simulink model "aavs1_8ap"  (R2013a)
settings: Solver=ode45  StartTime=0.0  StopTime=10.0  RelTol=1e-3
undefined symbols (not defined in the file or in its folder): sfp
libraries: xbsIndex_r4 x1437, casper_library_misc x32, xps_library x17
(part 3 of 11)

== system aavs1_8ap/eq/quant13 ==
  cin : Inport
  din : Inport  Port=2
  Delay{,1..3} (4 alike) : xbsIndex_r4/Delay  rst=off  infoeditControl=Selection of Reset will increase slice count due to use of real FFs and instead of SRLs  en=off  latency=1  dbl_ovrd=off  reg_retiming=off  block_type=delay
  Mult : xbsIndex_r4/Mult  precision=Full  arith_type="Signed  (2's comp)"  n_bits=16  bin_pt=14  quantization=Truncate  overflow=Wrap  en=off  latency=3  dbl_ovrd=off  use_behavioral_HDL=off  opt=Speed  use_embedded=on  optimum_pipeline=off  pipeline=on  use_rpm=on  placement_style=Triangular  block_type=mult
  Mult1 : xbsIndex_r4/Mult  precision=Full  arith_type="Signed  (2's comp)"  n_bits=16  bin_pt=14  quantization=Truncate  overflow=Wrap  en=off  latency=3  dbl_ovrd=off  use_behavioral_HDL=off  opt=Speed  use_embedded=on  optimum_pipeline=off  pipeline=on  use_rpm=on  placement_style=Triangular  block_type=mult
  and : xbsIndex_r4/Logical  logical_function=OR  inputs=2  en=off  latency=1  precision=Full  arith_type=Unsigned  n_bits=16  bin_pt=0  align_bp=on  dbl_ovrd=off  block_type=logical
  c_to_ri : casper_library_misc/c_to_ri  n_bits=18  bin_pt=17
  convert_of : Subsystem  AncestorBlock=casper_library_misc/convert_of  mask(convert_of){bit_width_i=16+18, binary_point_i=17+8, bit_width_o=8, binary_point_o=7, latency=3, adder_imp=DSP48, overflow=Saturate, quantization=Round  (unbiased: even values)}
      mask prompts: bit_width_i "Bit Width In"; binary_point_i "Binary Point In"; bit_width_o "Bit Width Out"; binary_point_o "Binary Point Out"; adder_imp "Adder Implementation"; overflow "Overflow Behaviour"; quantization "Quantization Behaviour"
      mask help:
      | Converts from one 2's complement bit-width
      | and/or binary point position to another.
      | Includes underflow/overflow indicator.
      mask init: same as aavs1_8ap/eq/quant/convert_of
      settings: AttributesFormatString=[34,25]->[8,7]
      mask TypeOptions adder_imp: Fabric | DSP48
      mask TypeOptions overflow: Wrap | Saturate | Error
      mask TypeOptions quantization: Truncate | Round  (unbiased: +/- Inf) | Round  (unbiased: even values)
  convert_of1 : Subsystem  AncestorBlock=casper_library_misc/convert_of  mask(convert_of){bit_width_i=16+18, binary_point_i=17+8, bit_width_o=8, binary_point_o=7, latency=3, adder_imp=DSP48, overflow=Saturate, quantization=Round  (unbiased: even values)}
      mask prompts: bit_width_i "Bit Width In"; binary_point_i "Binary Point In"; bit_width_o "Bit Width Out"; binary_point_o "Binary Point Out"; adder_imp "Adder Implementation"; overflow "Overflow Behaviour"; quantization "Quantization Behaviour"
      mask help:
      | Converts from one 2's complement bit-width
      | and/or binary point position to another.
      | Includes underflow/overflow indicator.
      mask init: same as aavs1_8ap/eq/quant/convert_of
      settings: AttributesFormatString=[34,25]->[8,7]
      mask TypeOptions adder_imp: Fabric | DSP48
      mask TypeOptions overflow: Wrap | Saturate | Error
      mask TypeOptions quantization: Truncate | Round  (unbiased: +/- Inf) | Round  (unbiased: even values)
  ri_to_c : casper_library_misc/ri_to_c
  symmetrize : Subsystem
  symmetrize1 : Subsystem
  dout : Outport
  of : Outport  Port=2
  wires:
  c_to_ri/2 -> Mult1/2
  c_to_ri/1 -> Mult/2
  symmetrize1/1(dout) -> ri_to_c/2
  symmetrize/1(dout) -> ri_to_c/1
  convert_of/1(dout) -> Delay2/1
  convert_of1/1(dout) -> Delay3/1
  Mult1/1 -> Delay/1
  convert_of1/2(of) -> and/2
  Mult/1 -> Delay1/1
  din/1 -> c_to_ri/1
  convert_of/2(of) -> and/1
  cin/1 -> Mult1/1, Mult/1
  and/1 -> of/1
  ri_to_c/1 -> dout/1
  Delay/1 -> convert_of1/1(din)
  Delay1/1 -> convert_of/1(din)
  Delay2/1 -> symmetrize/1(din)
  Delay3/1 -> symmetrize1/1(din)

== system aavs1_8ap/eq/quant14 ==
  cin : Inport
  din : Inport  Port=2
  Delay{,1..3} (4 alike) : xbsIndex_r4/Delay  rst=off  infoeditControl=Selection of Reset will increase slice count due to use of real FFs and instead of SRLs  en=off  latency=1  dbl_ovrd=off  reg_retiming=off  block_type=delay
  Mult : xbsIndex_r4/Mult  precision=Full  arith_type="Signed  (2's comp)"  n_bits=16  bin_pt=14  quantization=Truncate  overflow=Wrap  en=off  latency=3  dbl_ovrd=off  use_behavioral_HDL=off  opt=Speed  use_embedded=on  optimum_pipeline=off  pipeline=on  use_rpm=on  placement_style=Triangular  block_type=mult
  Mult1 : xbsIndex_r4/Mult  precision=Full  arith_type="Signed  (2's comp)"  n_bits=16  bin_pt=14  quantization=Truncate  overflow=Wrap  en=off  latency=3  dbl_ovrd=off  use_behavioral_HDL=off  opt=Speed  use_embedded=on  optimum_pipeline=off  pipeline=on  use_rpm=on  placement_style=Triangular  block_type=mult
  and : xbsIndex_r4/Logical  logical_function=OR  inputs=2  en=off  latency=1  precision=Full  arith_type=Unsigned  n_bits=16  bin_pt=0  align_bp=on  dbl_ovrd=off  block_type=logical
  c_to_ri : casper_library_misc/c_to_ri  n_bits=18  bin_pt=17
  convert_of : Subsystem  AncestorBlock=casper_library_misc/convert_of  mask(convert_of){bit_width_i=16+18, binary_point_i=17+8, bit_width_o=8, binary_point_o=7, latency=3, adder_imp=DSP48, overflow=Saturate, quantization=Round  (unbiased: even values)}
      mask prompts: bit_width_i "Bit Width In"; binary_point_i "Binary Point In"; bit_width_o "Bit Width Out"; binary_point_o "Binary Point Out"; adder_imp "Adder Implementation"; overflow "Overflow Behaviour"; quantization "Quantization Behaviour"
      mask help:
      | Converts from one 2's complement bit-width
      | and/or binary point position to another.
      | Includes underflow/overflow indicator.
      mask init: same as aavs1_8ap/eq/quant/convert_of
      settings: AttributesFormatString=[34,25]->[8,7]
      mask TypeOptions adder_imp: Fabric | DSP48
      mask TypeOptions overflow: Wrap | Saturate | Error
      mask TypeOptions quantization: Truncate | Round  (unbiased: +/- Inf) | Round  (unbiased: even values)
  convert_of1 : Subsystem  AncestorBlock=casper_library_misc/convert_of  mask(convert_of){bit_width_i=16+18, binary_point_i=17+8, bit_width_o=8, binary_point_o=7, latency=3, adder_imp=DSP48, overflow=Saturate, quantization=Round  (unbiased: even values)}
      mask prompts: bit_width_i "Bit Width In"; binary_point_i "Binary Point In"; bit_width_o "Bit Width Out"; binary_point_o "Binary Point Out"; adder_imp "Adder Implementation"; overflow "Overflow Behaviour"; quantization "Quantization Behaviour"
      mask help:
      | Converts from one 2's complement bit-width
      | and/or binary point position to another.
      | Includes underflow/overflow indicator.
      mask init: same as aavs1_8ap/eq/quant/convert_of
      settings: AttributesFormatString=[34,25]->[8,7]
      mask TypeOptions adder_imp: Fabric | DSP48
      mask TypeOptions overflow: Wrap | Saturate | Error
      mask TypeOptions quantization: Truncate | Round  (unbiased: +/- Inf) | Round  (unbiased: even values)
  ri_to_c : casper_library_misc/ri_to_c
  symmetrize : Subsystem
  symmetrize1 : Subsystem
  dout : Outport
  of : Outport  Port=2
  wires:
  Delay3/1 -> symmetrize1/1(din)
  Delay2/1 -> symmetrize/1(din)
  Delay1/1 -> convert_of/1(din)
  Delay/1 -> convert_of1/1(din)
  ri_to_c/1 -> dout/1
  and/1 -> of/1
  cin/1 -> Mult/1, Mult1/1
  convert_of/2(of) -> and/1
  din/1 -> c_to_ri/1
  Mult/1 -> Delay1/1
  convert_of1/2(of) -> and/2
  Mult1/1 -> Delay/1
  convert_of1/1(dout) -> Delay3/1
  convert_of/1(dout) -> Delay2/1
  symmetrize/1(dout) -> ri_to_c/1
  symmetrize1/1(dout) -> ri_to_c/2
  c_to_ri/1 -> Mult/2
  c_to_ri/2 -> Mult1/2

== system aavs1_8ap/eq/quant15 ==
  cin : Inport
  din : Inport  Port=2
  Delay{,1..3} (4 alike) : xbsIndex_r4/Delay  rst=off  infoeditControl=Selection of Reset will increase slice count due to use of real FFs and instead of SRLs  en=off  latency=1  dbl_ovrd=off  reg_retiming=off  block_type=delay
  Mult : xbsIndex_r4/Mult  precision=Full  arith_type="Signed  (2's comp)"  n_bits=16  bin_pt=14  quantization=Truncate  overflow=Wrap  en=off  latency=3  dbl_ovrd=off  use_behavioral_HDL=off  opt=Speed  use_embedded=on  optimum_pipeline=off  pipeline=on  use_rpm=on  placement_style=Triangular  block_type=mult
  Mult1 : xbsIndex_r4/Mult  precision=Full  arith_type="Signed  (2's comp)"  n_bits=16  bin_pt=14  quantization=Truncate  overflow=Wrap  en=off  latency=3  dbl_ovrd=off  use_behavioral_HDL=off  opt=Speed  use_embedded=on  optimum_pipeline=off  pipeline=on  use_rpm=on  placement_style=Triangular  block_type=mult
  and : xbsIndex_r4/Logical  logical_function=OR  inputs=2  en=off  latency=1  precision=Full  arith_type=Unsigned  n_bits=16  bin_pt=0  align_bp=on  dbl_ovrd=off  block_type=logical
  c_to_ri : casper_library_misc/c_to_ri  n_bits=18  bin_pt=17
  convert_of : Subsystem  AncestorBlock=casper_library_misc/convert_of  mask(convert_of){bit_width_i=16+18, binary_point_i=17+8, bit_width_o=8, binary_point_o=7, latency=3, adder_imp=DSP48, overflow=Saturate, quantization=Round  (unbiased: even values)}
      mask prompts: bit_width_i "Bit Width In"; binary_point_i "Binary Point In"; bit_width_o "Bit Width Out"; binary_point_o "Binary Point Out"; adder_imp "Adder Implementation"; overflow "Overflow Behaviour"; quantization "Quantization Behaviour"
      mask help:
      | Converts from one 2's complement bit-width
      | and/or binary point position to another.
      | Includes underflow/overflow indicator.
      mask init: same as aavs1_8ap/eq/quant/convert_of
      settings: AttributesFormatString=[34,25]->[8,7]
      mask TypeOptions adder_imp: Fabric | DSP48
      mask TypeOptions overflow: Wrap | Saturate | Error
      mask TypeOptions quantization: Truncate | Round  (unbiased: +/- Inf) | Round  (unbiased: even values)
  convert_of1 : Subsystem  AncestorBlock=casper_library_misc/convert_of  mask(convert_of){bit_width_i=16+18, binary_point_i=17+8, bit_width_o=8, binary_point_o=7, latency=3, adder_imp=DSP48, overflow=Saturate, quantization=Round  (unbiased: even values)}
      mask prompts: bit_width_i "Bit Width In"; binary_point_i "Binary Point In"; bit_width_o "Bit Width Out"; binary_point_o "Binary Point Out"; adder_imp "Adder Implementation"; overflow "Overflow Behaviour"; quantization "Quantization Behaviour"
      mask help:
      | Converts from one 2's complement bit-width
      | and/or binary point position to another.
      | Includes underflow/overflow indicator.
      mask init: same as aavs1_8ap/eq/quant/convert_of
      settings: AttributesFormatString=[34,25]->[8,7]
      mask TypeOptions adder_imp: Fabric | DSP48
      mask TypeOptions overflow: Wrap | Saturate | Error
      mask TypeOptions quantization: Truncate | Round  (unbiased: +/- Inf) | Round  (unbiased: even values)
  ri_to_c : casper_library_misc/ri_to_c
  symmetrize : Subsystem
  symmetrize1 : Subsystem
  dout : Outport
  of : Outport  Port=2
  wires:
  c_to_ri/2 -> Mult1/2
  c_to_ri/1 -> Mult/2
  symmetrize1/1(dout) -> ri_to_c/2
  symmetrize/1(dout) -> ri_to_c/1
  convert_of/1(dout) -> Delay2/1
  convert_of1/1(dout) -> Delay3/1
  Mult1/1 -> Delay/1
  convert_of1/2(of) -> and/2
  Mult/1 -> Delay1/1
  din/1 -> c_to_ri/1
  convert_of/2(of) -> and/1
  cin/1 -> Mult1/1, Mult/1
  and/1 -> of/1
  ri_to_c/1 -> dout/1
  Delay/1 -> convert_of1/1(din)
  Delay1/1 -> convert_of/1(din)
  Delay2/1 -> symmetrize/1(din)
  Delay3/1 -> symmetrize1/1(din)

== system aavs1_8ap/eq/quant2 ==
  cin : Inport
  din : Inport  Port=2
  Delay{,1..3} (4 alike) : xbsIndex_r4/Delay  rst=off  infoeditControl=Selection of Reset will increase slice count due to use of real FFs and instead of SRLs  en=off  latency=1  dbl_ovrd=off  reg_retiming=off  block_type=delay
  Mult : xbsIndex_r4/Mult  precision=Full  arith_type="Signed  (2's comp)"  n_bits=16  bin_pt=14  quantization=Truncate  overflow=Wrap  en=off  latency=3  dbl_ovrd=off  use_behavioral_HDL=off  opt=Speed  use_embedded=on  optimum_pipeline=off  pipeline=on  use_rpm=on  placement_style=Triangular  block_type=mult
  Mult1 : xbsIndex_r4/Mult  precision=Full  arith_type="Signed  (2's comp)"  n_bits=16  bin_pt=14  quantization=Truncate  overflow=Wrap  en=off  latency=3  dbl_ovrd=off  use_behavioral_HDL=off  opt=Speed  use_embedded=on  optimum_pipeline=off  pipeline=on  use_rpm=on  placement_style=Triangular  block_type=mult
  and : xbsIndex_r4/Logical  logical_function=OR  inputs=2  en=off  latency=1  precision=Full  arith_type=Unsigned  n_bits=16  bin_pt=0  align_bp=on  dbl_ovrd=off  block_type=logical
  c_to_ri : casper_library_misc/c_to_ri  n_bits=18  bin_pt=17
  convert_of : Subsystem  AncestorBlock=casper_library_misc/convert_of  mask(convert_of){bit_width_i=16+18, binary_point_i=17+8, bit_width_o=8, binary_point_o=7, latency=3, adder_imp=DSP48, overflow=Saturate, quantization=Round  (unbiased: even values)}
      mask prompts: bit_width_i "Bit Width In"; binary_point_i "Binary Point In"; bit_width_o "Bit Width Out"; binary_point_o "Binary Point Out"; adder_imp "Adder Implementation"; overflow "Overflow Behaviour"; quantization "Quantization Behaviour"
      mask help:
      | Converts from one 2's complement bit-width
      | and/or binary point position to another.
      | Includes underflow/overflow indicator.
      mask init: same as aavs1_8ap/eq/quant/convert_of
      settings: AttributesFormatString=[34,25]->[8,7]
      mask TypeOptions adder_imp: Fabric | DSP48
      mask TypeOptions overflow: Wrap | Saturate | Error
      mask TypeOptions quantization: Truncate | Round  (unbiased: +/- Inf) | Round  (unbiased: even values)
  convert_of1 : Subsystem  AncestorBlock=casper_library_misc/convert_of  mask(convert_of){bit_width_i=16+18, binary_point_i=17+8, bit_width_o=8, binary_point_o=7, latency=3, adder_imp=DSP48, overflow=Saturate, quantization=Round  (unbiased: even values)}
      mask prompts: bit_width_i "Bit Width In"; binary_point_i "Binary Point In"; bit_width_o "Bit Width Out"; binary_point_o "Binary Point Out"; adder_imp "Adder Implementation"; overflow "Overflow Behaviour"; quantization "Quantization Behaviour"
      mask help:
      | Converts from one 2's complement bit-width
      | and/or binary point position to another.
      | Includes underflow/overflow indicator.
      mask init: same as aavs1_8ap/eq/quant/convert_of
      settings: AttributesFormatString=[34,25]->[8,7]
      mask TypeOptions adder_imp: Fabric | DSP48
      mask TypeOptions overflow: Wrap | Saturate | Error
      mask TypeOptions quantization: Truncate | Round  (unbiased: +/- Inf) | Round  (unbiased: even values)
  ri_to_c : casper_library_misc/ri_to_c
  symmetrize : Subsystem
  symmetrize1 : Subsystem
  dout : Outport
  of : Outport  Port=2
  wires:
  c_to_ri/2 -> Mult1/2
  c_to_ri/1 -> Mult/2
  symmetrize1/1(dout) -> ri_to_c/2
  symmetrize/1(dout) -> ri_to_c/1
  convert_of/1(dout) -> Delay2/1
  convert_of1/1(dout) -> Delay3/1
  Mult1/1 -> Delay/1
  convert_of1/2(of) -> and/2
  Mult/1 -> Delay1/1
  din/1 -> c_to_ri/1
  convert_of/2(of) -> and/1
  cin/1 -> Mult1/1, Mult/1
  and/1 -> of/1
  ri_to_c/1 -> dout/1
  Delay/1 -> convert_of1/1(din)
  Delay1/1 -> convert_of/1(din)
  Delay2/1 -> symmetrize/1(din)
  Delay3/1 -> symmetrize1/1(din)

== system aavs1_8ap/eq/quant3 ==
  cin : Inport
  din : Inport  Port=2
  Delay{,1..3} (4 alike) : xbsIndex_r4/Delay  rst=off  infoeditControl=Selection of Reset will increase slice count due to use of real FFs and instead of SRLs  en=off  latency=1  dbl_ovrd=off  reg_retiming=off  block_type=delay
  Mult : xbsIndex_r4/Mult  precision=Full  arith_type="Signed  (2's comp)"  n_bits=16  bin_pt=14  quantization=Truncate  overflow=Wrap  en=off  latency=3  dbl_ovrd=off  use_behavioral_HDL=off  opt=Speed  use_embedded=on  optimum_pipeline=off  pipeline=on  use_rpm=on  placement_style=Triangular  block_type=mult
  Mult1 : xbsIndex_r4/Mult  precision=Full  arith_type="Signed  (2's comp)"  n_bits=16  bin_pt=14  quantization=Truncate  overflow=Wrap  en=off  latency=3  dbl_ovrd=off  use_behavioral_HDL=off  opt=Speed  use_embedded=on  optimum_pipeline=off  pipeline=on  use_rpm=on  placement_style=Triangular  block_type=mult
  and : xbsIndex_r4/Logical  logical_function=OR  inputs=2  en=off  latency=1  precision=Full  arith_type=Unsigned  n_bits=16  bin_pt=0  align_bp=on  dbl_ovrd=off  block_type=logical
  c_to_ri : casper_library_misc/c_to_ri  n_bits=18  bin_pt=17
  convert_of : Subsystem  AncestorBlock=casper_library_misc/convert_of  mask(convert_of){bit_width_i=16+18, binary_point_i=17+8, bit_width_o=8, binary_point_o=7, latency=3, adder_imp=DSP48, overflow=Saturate, quantization=Round  (unbiased: even values)}
      mask prompts: bit_width_i "Bit Width In"; binary_point_i "Binary Point In"; bit_width_o "Bit Width Out"; binary_point_o "Binary Point Out"; adder_imp "Adder Implementation"; overflow "Overflow Behaviour"; quantization "Quantization Behaviour"
      mask help:
      | Converts from one 2's complement bit-width
      | and/or binary point position to another.
      | Includes underflow/overflow indicator.
      mask init: same as aavs1_8ap/eq/quant/convert_of
      settings: AttributesFormatString=[34,25]->[8,7]
      mask TypeOptions adder_imp: Fabric | DSP48
      mask TypeOptions overflow: Wrap | Saturate | Error
      mask TypeOptions quantization: Truncate | Round  (unbiased: +/- Inf) | Round  (unbiased: even values)
  convert_of1 : Subsystem  AncestorBlock=casper_library_misc/convert_of  mask(convert_of){bit_width_i=16+18, binary_point_i=17+8, bit_width_o=8, binary_point_o=7, latency=3, adder_imp=DSP48, overflow=Saturate, quantization=Round  (unbiased: even values)}
      mask prompts: bit_width_i "Bit Width In"; binary_point_i "Binary Point In"; bit_width_o "Bit Width Out"; binary_point_o "Binary Point Out"; adder_imp "Adder Implementation"; overflow "Overflow Behaviour"; quantization "Quantization Behaviour"
      mask help:
      | Converts from one 2's complement bit-width
      | and/or binary point position to another.
      | Includes underflow/overflow indicator.
      mask init: same as aavs1_8ap/eq/quant/convert_of
      settings: AttributesFormatString=[34,25]->[8,7]
      mask TypeOptions adder_imp: Fabric | DSP48
      mask TypeOptions overflow: Wrap | Saturate | Error
      mask TypeOptions quantization: Truncate | Round  (unbiased: +/- Inf) | Round  (unbiased: even values)
  ri_to_c : casper_library_misc/ri_to_c
  symmetrize : Subsystem
  symmetrize1 : Subsystem
  dout : Outport
  of : Outport  Port=2
  wires:
  Delay3/1 -> symmetrize1/1(din)
  Delay2/1 -> symmetrize/1(din)
  Delay1/1 -> convert_of/1(din)
  Delay/1 -> convert_of1/1(din)
  ri_to_c/1 -> dout/1
  and/1 -> of/1
  cin/1 -> Mult/1, Mult1/1
  convert_of/2(of) -> and/1
  din/1 -> c_to_ri/1
  Mult/1 -> Delay1/1
  convert_of1/2(of) -> and/2
  Mult1/1 -> Delay/1
  convert_of1/1(dout) -> Delay3/1
  convert_of/1(dout) -> Delay2/1
  symmetrize/1(dout) -> ri_to_c/1
  symmetrize1/1(dout) -> ri_to_c/2
  c_to_ri/1 -> Mult/2
  c_to_ri/2 -> Mult1/2

== system aavs1_8ap/eq/quant4 ==
  cin : Inport
  din : Inport  Port=2
  Delay{,1..3} (4 alike) : xbsIndex_r4/Delay  rst=off  infoeditControl=Selection of Reset will increase slice count due to use of real FFs and instead of SRLs  en=off  latency=1  dbl_ovrd=off  reg_retiming=off  block_type=delay
  Mult : xbsIndex_r4/Mult  precision=Full  arith_type="Signed  (2's comp)"  n_bits=16  bin_pt=14  quantization=Truncate  overflow=Wrap  en=off  latency=3  dbl_ovrd=off  use_behavioral_HDL=off  opt=Speed  use_embedded=on  optimum_pipeline=off  pipeline=on  use_rpm=on  placement_style=Triangular  block_type=mult
  Mult1 : xbsIndex_r4/Mult  precision=Full  arith_type="Signed  (2's comp)"  n_bits=16  bin_pt=14  quantization=Truncate  overflow=Wrap  en=off  latency=3  dbl_ovrd=off  use_behavioral_HDL=off  opt=Speed  use_embedded=on  optimum_pipeline=off  pipeline=on  use_rpm=on  placement_style=Triangular  block_type=mult
  and : xbsIndex_r4/Logical  logical_function=OR  inputs=2  en=off  latency=1  precision=Full  arith_type=Unsigned  n_bits=16  bin_pt=0  align_bp=on  dbl_ovrd=off  block_type=logical
  c_to_ri : casper_library_misc/c_to_ri  n_bits=18  bin_pt=17
  convert_of : Subsystem  AncestorBlock=casper_library_misc/convert_of  mask(convert_of){bit_width_i=16+18, binary_point_i=17+8, bit_width_o=8, binary_point_o=7, latency=3, adder_imp=DSP48, overflow=Saturate, quantization=Round  (unbiased: even values)}
      mask prompts: bit_width_i "Bit Width In"; binary_point_i "Binary Point In"; bit_width_o "Bit Width Out"; binary_point_o "Binary Point Out"; adder_imp "Adder Implementation"; overflow "Overflow Behaviour"; quantization "Quantization Behaviour"
      mask help:
      | Converts from one 2's complement bit-width
      | and/or binary point position to another.
      | Includes underflow/overflow indicator.
      mask init: same as aavs1_8ap/eq/quant/convert_of
      settings: AttributesFormatString=[34,25]->[8,7]
      mask TypeOptions adder_imp: Fabric | DSP48
      mask TypeOptions overflow: Wrap | Saturate | Error
      mask TypeOptions quantization: Truncate | Round  (unbiased: +/- Inf) | Round  (unbiased: even values)
  convert_of1 : Subsystem  AncestorBlock=casper_library_misc/convert_of  mask(convert_of){bit_width_i=16+18, binary_point_i=17+8, bit_width_o=8, binary_point_o=7, latency=3, adder_imp=DSP48, overflow=Saturate, quantization=Round  (unbiased: even values)}
      mask prompts: bit_width_i "Bit Width In"; binary_point_i "Binary Point In"; bit_width_o "Bit Width Out"; binary_point_o "Binary Point Out"; adder_imp "Adder Implementation"; overflow "Overflow Behaviour"; quantization "Quantization Behaviour"
      mask help:
      | Converts from one 2's complement bit-width
      | and/or binary point position to another.
      | Includes underflow/overflow indicator.
      mask init: same as aavs1_8ap/eq/quant/convert_of
      settings: AttributesFormatString=[34,25]->[8,7]
      mask TypeOptions adder_imp: Fabric | DSP48
      mask TypeOptions overflow: Wrap | Saturate | Error
      mask TypeOptions quantization: Truncate | Round  (unbiased: +/- Inf) | Round  (unbiased: even values)
  ri_to_c : casper_library_misc/ri_to_c
  symmetrize : Subsystem
  symmetrize1 : Subsystem
  dout : Outport
  of : Outport  Port=2
  wires:
  Delay3/1 -> symmetrize1/1(din)
  Delay2/1 -> symmetrize/1(din)
  Delay1/1 -> convert_of/1(din)
  Delay/1 -> convert_of1/1(din)
  ri_to_c/1 -> dout/1
  and/1 -> of/1
  cin/1 -> Mult/1, Mult1/1
  convert_of/2(of) -> and/1
  din/1 -> c_to_ri/1
  Mult/1 -> Delay1/1
  convert_of1/2(of) -> and/2
  Mult1/1 -> Delay/1
  convert_of1/1(dout) -> Delay3/1
  convert_of/1(dout) -> Delay2/1
  symmetrize/1(dout) -> ri_to_c/1
  symmetrize1/1(dout) -> ri_to_c/2
  c_to_ri/1 -> Mult/2
  c_to_ri/2 -> Mult1/2

== system aavs1_8ap/eq/quant5 ==
  cin : Inport
  din : Inport  Port=2
  Delay{,1..3} (4 alike) : xbsIndex_r4/Delay  rst=off  infoeditControl=Selection of Reset will increase slice count due to use of real FFs and instead of SRLs  en=off  latency=1  dbl_ovrd=off  reg_retiming=off  block_type=delay
  Mult : xbsIndex_r4/Mult  precision=Full  arith_type="Signed  (2's comp)"  n_bits=16  bin_pt=14  quantization=Truncate  overflow=Wrap  en=off  latency=3  dbl_ovrd=off  use_behavioral_HDL=off  opt=Speed  use_embedded=on  optimum_pipeline=off  pipeline=on  use_rpm=on  placement_style=Triangular  block_type=mult
  Mult1 : xbsIndex_r4/Mult  precision=Full  arith_type="Signed  (2's comp)"  n_bits=16  bin_pt=14  quantization=Truncate  overflow=Wrap  en=off  latency=3  dbl_ovrd=off  use_behavioral_HDL=off  opt=Speed  use_embedded=on  optimum_pipeline=off  pipeline=on  use_rpm=on  placement_style=Triangular  block_type=mult
  and : xbsIndex_r4/Logical  logical_function=OR  inputs=2  en=off  latency=1  precision=Full  arith_type=Unsigned  n_bits=16  bin_pt=0  align_bp=on  dbl_ovrd=off  block_type=logical
  c_to_ri : casper_library_misc/c_to_ri  n_bits=18  bin_pt=17
  convert_of : Subsystem  AncestorBlock=casper_library_misc/convert_of  mask(convert_of){bit_width_i=16+18, binary_point_i=17+8, bit_width_o=8, binary_point_o=7, latency=3, adder_imp=DSP48, overflow=Saturate, quantization=Round  (unbiased: even values)}
      mask prompts: bit_width_i "Bit Width In"; binary_point_i "Binary Point In"; bit_width_o "Bit Width Out"; binary_point_o "Binary Point Out"; adder_imp "Adder Implementation"; overflow "Overflow Behaviour"; quantization "Quantization Behaviour"
      mask help:
      | Converts from one 2's complement bit-width
      | and/or binary point position to another.
      | Includes underflow/overflow indicator.
      mask init: same as aavs1_8ap/eq/quant/convert_of
      settings: AttributesFormatString=[34,25]->[8,7]
      mask TypeOptions adder_imp: Fabric | DSP48
      mask TypeOptions overflow: Wrap | Saturate | Error
      mask TypeOptions quantization: Truncate | Round  (unbiased: +/- Inf) | Round  (unbiased: even values)
  convert_of1 : Subsystem  AncestorBlock=casper_library_misc/convert_of  mask(convert_of){bit_width_i=16+18, binary_point_i=17+8, bit_width_o=8, binary_point_o=7, latency=3, adder_imp=DSP48, overflow=Saturate, quantization=Round  (unbiased: even values)}
      mask prompts: bit_width_i "Bit Width In"; binary_point_i "Binary Point In"; bit_width_o "Bit Width Out"; binary_point_o "Binary Point Out"; adder_imp "Adder Implementation"; overflow "Overflow Behaviour"; quantization "Quantization Behaviour"
      mask help:
      | Converts from one 2's complement bit-width
      | and/or binary point position to another.
      | Includes underflow/overflow indicator.
      mask init: same as aavs1_8ap/eq/quant/convert_of
      settings: AttributesFormatString=[34,25]->[8,7]
      mask TypeOptions adder_imp: Fabric | DSP48
      mask TypeOptions overflow: Wrap | Saturate | Error
      mask TypeOptions quantization: Truncate | Round  (unbiased: +/- Inf) | Round  (unbiased: even values)
  ri_to_c : casper_library_misc/ri_to_c
  symmetrize : Subsystem
  symmetrize1 : Subsystem
  dout : Outport
  of : Outport  Port=2
  wires:
  c_to_ri/2 -> Mult1/2
  c_to_ri/1 -> Mult/2
  symmetrize1/1(dout) -> ri_to_c/2
  symmetrize/1(dout) -> ri_to_c/1
  convert_of/1(dout) -> Delay2/1
  convert_of1/1(dout) -> Delay3/1
  Mult1/1 -> Delay/1
  convert_of1/2(of) -> and/2
  Mult/1 -> Delay1/1
  din/1 -> c_to_ri/1
  convert_of/2(of) -> and/1
  cin/1 -> Mult1/1, Mult/1
  and/1 -> of/1
  ri_to_c/1 -> dout/1
  Delay/1 -> convert_of1/1(din)
  Delay1/1 -> convert_of/1(din)
  Delay2/1 -> symmetrize/1(din)
  Delay3/1 -> symmetrize1/1(din)

== system aavs1_8ap/eq/quant6 ==
  cin : Inport
  din : Inport  Port=2
  Delay{,1..3} (4 alike) : xbsIndex_r4/Delay  rst=off  infoeditControl=Selection of Reset will increase slice count due to use of real FFs and instead of SRLs  en=off  latency=1  dbl_ovrd=off  reg_retiming=off  block_type=delay
  Mult : xbsIndex_r4/Mult  precision=Full  arith_type="Signed  (2's comp)"  n_bits=16  bin_pt=14  quantization=Truncate  overflow=Wrap  en=off  latency=3  dbl_ovrd=off  use_behavioral_HDL=off  opt=Speed  use_embedded=on  optimum_pipeline=off  pipeline=on  use_rpm=on  placement_style=Triangular  block_type=mult
  Mult1 : xbsIndex_r4/Mult  precision=Full  arith_type="Signed  (2's comp)"  n_bits=16  bin_pt=14  quantization=Truncate  overflow=Wrap  en=off  latency=3  dbl_ovrd=off  use_behavioral_HDL=off  opt=Speed  use_embedded=on  optimum_pipeline=off  pipeline=on  use_rpm=on  placement_style=Triangular  block_type=mult
  and : xbsIndex_r4/Logical  logical_function=OR  inputs=2  en=off  latency=1  precision=Full  arith_type=Unsigned  n_bits=16  bin_pt=0  align_bp=on  dbl_ovrd=off  block_type=logical
  c_to_ri : casper_library_misc/c_to_ri  n_bits=18  bin_pt=17
  convert_of : Subsystem  AncestorBlock=casper_library_misc/convert_of  mask(convert_of){bit_width_i=16+18, binary_point_i=17+8, bit_width_o=8, binary_point_o=7, latency=3, adder_imp=DSP48, overflow=Saturate, quantization=Round  (unbiased: even values)}
      mask prompts: bit_width_i "Bit Width In"; binary_point_i "Binary Point In"; bit_width_o "Bit Width Out"; binary_point_o "Binary Point Out"; adder_imp "Adder Implementation"; overflow "Overflow Behaviour"; quantization "Quantization Behaviour"
      mask help:
      | Converts from one 2's complement bit-width
      | and/or binary point position to another.
      | Includes underflow/overflow indicator.
      mask init: same as aavs1_8ap/eq/quant/convert_of
      settings: AttributesFormatString=[34,25]->[8,7]
      mask TypeOptions adder_imp: Fabric | DSP48
      mask TypeOptions overflow: Wrap | Saturate | Error
      mask TypeOptions quantization: Truncate | Round  (unbiased: +/- Inf) | Round  (unbiased: even values)
  convert_of1 : Subsystem  AncestorBlock=casper_library_misc/convert_of  mask(convert_of){bit_width_i=16+18, binary_point_i=17+8, bit_width_o=8, binary_point_o=7, latency=3, adder_imp=DSP48, overflow=Saturate, quantization=Round  (unbiased: even values)}
      mask prompts: bit_width_i "Bit Width In"; binary_point_i "Binary Point In"; bit_width_o "Bit Width Out"; binary_point_o "Binary Point Out"; adder_imp "Adder Implementation"; overflow "Overflow Behaviour"; quantization "Quantization Behaviour"
      mask help:
      | Converts from one 2's complement bit-width
      | and/or binary point position to another.
      | Includes underflow/overflow indicator.
      mask init: same as aavs1_8ap/eq/quant/convert_of
      settings: AttributesFormatString=[34,25]->[8,7]
      mask TypeOptions adder_imp: Fabric | DSP48
      mask TypeOptions overflow: Wrap | Saturate | Error
      mask TypeOptions quantization: Truncate | Round  (unbiased: +/- Inf) | Round  (unbiased: even values)
  ri_to_c : casper_library_misc/ri_to_c
  symmetrize : Subsystem
  symmetrize1 : Subsystem
  dout : Outport
  of : Outport  Port=2
  wires:
  Delay3/1 -> symmetrize1/1(din)
  Delay2/1 -> symmetrize/1(din)
  Delay1/1 -> convert_of/1(din)
  Delay/1 -> convert_of1/1(din)
  ri_to_c/1 -> dout/1
  and/1 -> of/1
  cin/1 -> Mult/1, Mult1/1
  convert_of/2(of) -> and/1
  din/1 -> c_to_ri/1
  Mult/1 -> Delay1/1
  convert_of1/2(of) -> and/2
  Mult1/1 -> Delay/1
  convert_of1/1(dout) -> Delay3/1
  convert_of/1(dout) -> Delay2/1
  symmetrize/1(dout) -> ri_to_c/1
  symmetrize1/1(dout) -> ri_to_c/2
  c_to_ri/1 -> Mult/2
  c_to_ri/2 -> Mult1/2

== system aavs1_8ap/eq/quant7 ==
  cin : Inport
  din : Inport  Port=2
  Delay{,1..3} (4 alike) : xbsIndex_r4/Delay  rst=off  infoeditControl=Selection of Reset will increase slice count due to use of real FFs and instead of SRLs  en=off  latency=1  dbl_ovrd=off  reg_retiming=off  block_type=delay
  Mult : xbsIndex_r4/Mult  precision=Full  arith_type="Signed  (2's comp)"  n_bits=16  bin_pt=14  quantization=Truncate  overflow=Wrap  en=off  latency=3  dbl_ovrd=off  use_behavioral_HDL=off  opt=Speed  use_embedded=on  optimum_pipeline=off  pipeline=on  use_rpm=on  placement_style=Triangular  block_type=mult
  Mult1 : xbsIndex_r4/Mult  precision=Full  arith_type="Signed  (2's comp)"  n_bits=16  bin_pt=14  quantization=Truncate  overflow=Wrap  en=off  latency=3  dbl_ovrd=off  use_behavioral_HDL=off  opt=Speed  use_embedded=on  optimum_pipeline=off  pipeline=on  use_rpm=on  placement_style=Triangular  block_type=mult
  and : xbsIndex_r4/Logical  logical_function=OR  inputs=2  en=off  latency=1  precision=Full  arith_type=Unsigned  n_bits=16  bin_pt=0  align_bp=on  dbl_ovrd=off  block_type=logical
  c_to_ri : casper_library_misc/c_to_ri  n_bits=18  bin_pt=17
  convert_of : Subsystem  AncestorBlock=casper_library_misc/convert_of  mask(convert_of){bit_width_i=16+18, binary_point_i=17+8, bit_width_o=8, binary_point_o=7, latency=3, adder_imp=DSP48, overflow=Saturate, quantization=Round  (unbiased: even values)}
      mask prompts: bit_width_i "Bit Width In"; binary_point_i "Binary Point In"; bit_width_o "Bit Width Out"; binary_point_o "Binary Point Out"; adder_imp "Adder Implementation"; overflow "Overflow Behaviour"; quantization "Quantization Behaviour"
      mask help:
      | Converts from one 2's complement bit-width
      | and/or binary point position to another.
      | Includes underflow/overflow indicator.
      mask init: same as aavs1_8ap/eq/quant/convert_of
      settings: AttributesFormatString=[34,25]->[8,7]
      mask TypeOptions adder_imp: Fabric | DSP48
      mask TypeOptions overflow: Wrap | Saturate | Error
      mask TypeOptions quantization: Truncate | Round  (unbiased: +/- Inf) | Round  (unbiased: even values)
  convert_of1 : Subsystem  AncestorBlock=casper_library_misc/convert_of  mask(convert_of){bit_width_i=16+18, binary_point_i=17+8, bit_width_o=8, binary_point_o=7, latency=3, adder_imp=DSP48, overflow=Saturate, quantization=Round  (unbiased: even values)}
      mask prompts: bit_width_i "Bit Width In"; binary_point_i "Binary Point In"; bit_width_o "Bit Width Out"; binary_point_o "Binary Point Out"; adder_imp "Adder Implementation"; overflow "Overflow Behaviour"; quantization "Quantization Behaviour"
      mask help:
      | Converts from one 2's complement bit-width
      | and/or binary point position to another.
      | Includes underflow/overflow indicator.
      mask init: same as aavs1_8ap/eq/quant/convert_of
      settings: AttributesFormatString=[34,25]->[8,7]
      mask TypeOptions adder_imp: Fabric | DSP48
      mask TypeOptions overflow: Wrap | Saturate | Error
      mask TypeOptions quantization: Truncate | Round  (unbiased: +/- Inf) | Round  (unbiased: even values)
  ri_to_c : casper_library_misc/ri_to_c
  symmetrize : Subsystem
  symmetrize1 : Subsystem
  dout : Outport
  of : Outport  Port=2
  wires:
  c_to_ri/2 -> Mult1/2
  c_to_ri/1 -> Mult/2
  symmetrize1/1(dout) -> ri_to_c/2
  symmetrize/1(dout) -> ri_to_c/1
  convert_of/1(dout) -> Delay2/1
  convert_of1/1(dout) -> Delay3/1
  Mult1/1 -> Delay/1
  convert_of1/2(of) -> and/2
  Mult/1 -> Delay1/1
  din/1 -> c_to_ri/1
  convert_of/2(of) -> and/1
  cin/1 -> Mult1/1, Mult/1
  and/1 -> of/1
  ri_to_c/1 -> dout/1
  Delay/1 -> convert_of1/1(din)
  Delay1/1 -> convert_of/1(din)
  Delay2/1 -> symmetrize/1(din)
  Delay3/1 -> symmetrize1/1(din)

== system aavs1_8ap/eq/quant8 ==
  cin : Inport
  din : Inport  Port=2
  Delay{,1..3} (4 alike) : xbsIndex_r4/Delay  rst=off  infoeditControl=Selection of Reset will increase slice count due to use of real FFs and instead of SRLs  en=off  latency=1  dbl_ovrd=off  reg_retiming=off  block_type=delay
  Mult : xbsIndex_r4/Mult  precision=Full  arith_type="Signed  (2's comp)"  n_bits=16  bin_pt=14  quantization=Truncate  overflow=Wrap  en=off  latency=3  dbl_ovrd=off  use_behavioral_HDL=off  opt=Speed  use_embedded=on  optimum_pipeline=off  pipeline=on  use_rpm=on  placement_style=Triangular  block_type=mult
  Mult1 : xbsIndex_r4/Mult  precision=Full  arith_type="Signed  (2's comp)"  n_bits=16  bin_pt=14  quantization=Truncate  overflow=Wrap  en=off  latency=3  dbl_ovrd=off  use_behavioral_HDL=off  opt=Speed  use_embedded=on  optimum_pipeline=off  pipeline=on  use_rpm=on  placement_style=Triangular  block_type=mult
  and : xbsIndex_r4/Logical  logical_function=OR  inputs=2  en=off  latency=1  precision=Full  arith_type=Unsigned  n_bits=16  bin_pt=0  align_bp=on  dbl_ovrd=off  block_type=logical
  c_to_ri : casper_library_misc/c_to_ri  n_bits=18  bin_pt=17
  convert_of : Subsystem  AncestorBlock=casper_library_misc/convert_of  mask(convert_of){bit_width_i=16+18, binary_point_i=17+8, bit_width_o=8, binary_point_o=7, latency=3, adder_imp=DSP48, overflow=Saturate, quantization=Round  (unbiased: even values)}
      mask prompts: bit_width_i "Bit Width In"; binary_point_i "Binary Point In"; bit_width_o "Bit Width Out"; binary_point_o "Binary Point Out"; adder_imp "Adder Implementation"; overflow "Overflow Behaviour"; quantization "Quantization Behaviour"
      mask help:
      | Converts from one 2's complement bit-width
      | and/or binary point position to another.
      | Includes underflow/overflow indicator.
      mask init: same as aavs1_8ap/eq/quant/convert_of
      settings: AttributesFormatString=[34,25]->[8,7]
      mask TypeOptions adder_imp: Fabric | DSP48
      mask TypeOptions overflow: Wrap | Saturate | Error
      mask TypeOptions quantization: Truncate | Round  (unbiased: +/- Inf) | Round  (unbiased: even values)
  convert_of1 : Subsystem  AncestorBlock=casper_library_misc/convert_of  mask(convert_of){bit_width_i=16+18, binary_point_i=17+8, bit_width_o=8, binary_point_o=7, latency=3, adder_imp=DSP48, overflow=Saturate, quantization=Round  (unbiased: even values)}
      mask prompts: bit_width_i "Bit Width In"; binary_point_i "Binary Point In"; bit_width_o "Bit Width Out"; binary_point_o "Binary Point Out"; adder_imp "Adder Implementation"; overflow "Overflow Behaviour"; quantization "Quantization Behaviour"
      mask help:
      | Converts from one 2's complement bit-width
      | and/or binary point position to another.
      | Includes underflow/overflow indicator.
      mask init: same as aavs1_8ap/eq/quant/convert_of
      settings: AttributesFormatString=[34,25]->[8,7]
      mask TypeOptions adder_imp: Fabric | DSP48
      mask TypeOptions overflow: Wrap | Saturate | Error
      mask TypeOptions quantization: Truncate | Round  (unbiased: +/- Inf) | Round  (unbiased: even values)
  ri_to_c : casper_library_misc/ri_to_c
  symmetrize : Subsystem
  symmetrize1 : Subsystem
  dout : Outport
  of : Outport  Port=2
  wires:
  c_to_ri/2 -> Mult1/2
  c_to_ri/1 -> Mult/2
  symmetrize1/1(dout) -> ri_to_c/2
  symmetrize/1(dout) -> ri_to_c/1
  convert_of/1(dout) -> Delay2/1
  convert_of1/1(dout) -> Delay3/1
  Mult1/1 -> Delay/1
  convert_of1/2(of) -> and/2
  Mult/1 -> Delay1/1
  din/1 -> c_to_ri/1
  convert_of/2(of) -> and/1
  cin/1 -> Mult1/1, Mult/1
  and/1 -> of/1
  ri_to_c/1 -> dout/1
  Delay/1 -> convert_of1/1(din)
  Delay1/1 -> convert_of/1(din)
  Delay2/1 -> symmetrize/1(din)
  Delay3/1 -> symmetrize1/1(din)

== system aavs1_8ap/eq/quant9 ==
  cin : Inport
  din : Inport  Port=2
  Delay{,1..3} (4 alike) : xbsIndex_r4/Delay  rst=off  infoeditControl=Selection of Reset will increase slice count due to use of real FFs and instead of SRLs  en=off  latency=1  dbl_ovrd=off  reg_retiming=off  block_type=delay
  Mult : xbsIndex_r4/Mult  precision=Full  arith_type="Signed  (2's comp)"  n_bits=16  bin_pt=14  quantization=Truncate  overflow=Wrap  en=off  latency=3  dbl_ovrd=off  use_behavioral_HDL=off  opt=Speed  use_embedded=on  optimum_pipeline=off  pipeline=on  use_rpm=on  placement_style=Triangular  block_type=mult
  Mult1 : xbsIndex_r4/Mult  precision=Full  arith_type="Signed  (2's comp)"  n_bits=16  bin_pt=14  quantization=Truncate  overflow=Wrap  en=off  latency=3  dbl_ovrd=off  use_behavioral_HDL=off  opt=Speed  use_embedded=on  optimum_pipeline=off  pipeline=on  use_rpm=on  placement_style=Triangular  block_type=mult
  and : xbsIndex_r4/Logical  logical_function=OR  inputs=2  en=off  latency=1  precision=Full  arith_type=Unsigned  n_bits=16  bin_pt=0  align_bp=on  dbl_ovrd=off  block_type=logical
  c_to_ri : casper_library_misc/c_to_ri  n_bits=18  bin_pt=17
  convert_of : Subsystem  AncestorBlock=casper_library_misc/convert_of  mask(convert_of){bit_width_i=16+18, binary_point_i=17+8, bit_width_o=8, binary_point_o=7, latency=3, adder_imp=DSP48, overflow=Saturate, quantization=Round  (unbiased: even values)}
      mask prompts: bit_width_i "Bit Width In"; binary_point_i "Binary Point In"; bit_width_o "Bit Width Out"; binary_point_o "Binary Point Out"; adder_imp "Adder Implementation"; overflow "Overflow Behaviour"; quantization "Quantization Behaviour"
      mask help:
      | Converts from one 2's complement bit-width
      | and/or binary point position to another.
      | Includes underflow/overflow indicator.
      mask init: same as aavs1_8ap/eq/quant/convert_of
      settings: AttributesFormatString=[34,25]->[8,7]
      mask TypeOptions adder_imp: Fabric | DSP48
      mask TypeOptions overflow: Wrap | Saturate | Error
      mask TypeOptions quantization: Truncate | Round  (unbiased: +/- Inf) | Round  (unbiased: even values)
  convert_of1 : Subsystem  AncestorBlock=casper_library_misc/convert_of  mask(convert_of){bit_width_i=16+18, binary_point_i=17+8, bit_width_o=8, binary_point_o=7, latency=3, adder_imp=DSP48, overflow=Saturate, quantization=Round  (unbiased: even values)}
      mask prompts: bit_width_i "Bit Width In"; binary_point_i "Binary Point In"; bit_width_o "Bit Width Out"; binary_point_o "Binary Point Out"; adder_imp "Adder Implementation"; overflow "Overflow Behaviour"; quantization "Quantization Behaviour"
      mask help:
      | Converts from one 2's complement bit-width
      | and/or binary point position to another.
      | Includes underflow/overflow indicator.
      mask init: same as aavs1_8ap/eq/quant/convert_of
      settings: AttributesFormatString=[34,25]->[8,7]
      mask TypeOptions adder_imp: Fabric | DSP48
      mask TypeOptions overflow: Wrap | Saturate | Error
      mask TypeOptions quantization: Truncate | Round  (unbiased: +/- Inf) | Round  (unbiased: even values)
  ri_to_c : casper_library_misc/ri_to_c
  symmetrize : Subsystem
  symmetrize1 : Subsystem
  dout : Outport
  of : Outport  Port=2
  wires:
  Delay3/1 -> symmetrize1/1(din)
  Delay2/1 -> symmetrize/1(din)
  Delay1/1 -> convert_of/1(din)
  Delay/1 -> convert_of1/1(din)
  ri_to_c/1 -> dout/1
  and/1 -> of/1
  cin/1 -> Mult/1, Mult1/1
  convert_of/2(of) -> and/1
  din/1 -> c_to_ri/1
  Mult/1 -> Delay1/1
  convert_of1/2(of) -> and/2
  Mult1/1 -> Delay/1
  convert_of1/1(dout) -> Delay3/1
  convert_of/1(dout) -> Delay2/1
  symmetrize/1(dout) -> ri_to_c/1
  symmetrize1/1(dout) -> ri_to_c/2
  c_to_ri/1 -> Mult/2
  c_to_ri/2 -> Mult1/2

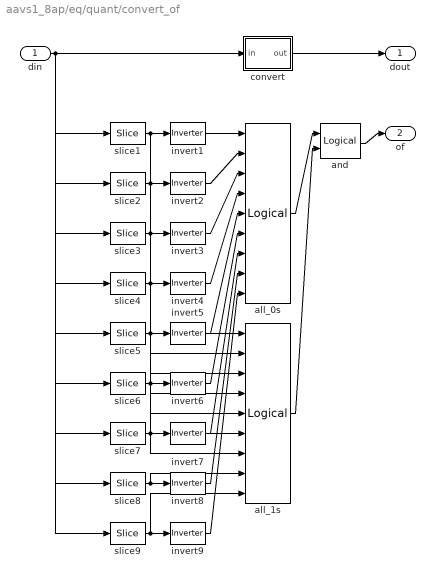
== system aavs1_8ap/eq/quant/convert_of ==
  din : Inport
  all_0s : xbsIndex_r4/Logical  logical_function=NAND  inputs=9  en=off  latency=latency  precision=Full  arith_type=Unsigned  n_bits=16  bin_pt=0  align_bp=on  dbl_ovrd=off  block_type=logical
  all_1s : xbsIndex_r4/Logical  logical_function=NAND  inputs=9  en=off  latency=latency  precision=Full  arith_type=Unsigned  n_bits=16  bin_pt=0  align_bp=on  dbl_ovrd=off  block_type=logical
  and : xbsIndex_r4/Logical  logical_function=AND  inputs=2  en=off  latency=0  precision=Full  arith_type=Unsigned  n_bits=16  bin_pt=0  align_bp=on  dbl_ovrd=off  block_type=logical
  convert : Subsystem  AncestorBlock=casper_library_misc/convert  mask(convert){bin_pt_in=binary_point_i, n_bits_out=bit_width_o, bin_pt_out=binary_point_o, quantization=Round  (unbiased: Even Values), overflow=Saturate, latency=latency, adder_imp=DSP48}
      mask prompts: bin_pt_in "Binary Point In"; n_bits_out "Bit Width Out"; bin_pt_out "Binary Point Out"; adder_imp "Adder Implementation"
      mask help:
      | Convert input value to the specified bit width and precision.
      |
      | Does not support upscaling number of fractional bits (eg 8_5 to 8_4 is ok, but not 8_4 to 8_5).
      mask init:
      | convert_init(gcb, ...
      |     'bin_pt_in',bin_pt_in, ...
      |     'n_bits_out',n_bits_out,...
      |     'bin_pt_out',bin_pt_out, ...
      |     'quantization',quantization,...
      |     'overflow',overflow,...
      |     'latency',latency,...
      |     'adder_imp',adder_imp);
      settings: AttributesFormatString=|
      | N_25 ==> 8_7
      | round even, saturate
      | latency = 3
      mask Help:
      | <pre>
      | Description::
      | 
      | Outputs converted version of the input.
      | 
      | Mask Parameters::
      | 
      | Binary Point In (bin_pt_in): Specifies the binary point location in the input.
      | 
      | Bit Width Out (n_bits_out): Specifies the width of the output.
      | 
      | Binary Point Out (bin_pt_out): Specifies the binary point location in the output.
      | 
      | Quantization (quantization): Specifies quantization handling.
      | 
      | Overflow (overflow): Specifies overflow handling.
      | 
      | Latency (latency): Specifies the latency of the underlying adder block, which is the overall
      | latency of this block as well.
      | Adder Implementation (adder_imp) specifies whether the adder should be implemented in DSP or logic. In either case, pipelining is enabled.</pre>
      mask TypeOptions quantization: Truncate | Round  (unbiased: +/- Inf) | Round  (unbiased: Even Values) | Round  (unbiased: Zero) | Round  (unbiased: Odd Values) | Round  (biased: Up) | Round  (biased: Down)
      mask TypeOptions overflow: Wrap | Saturate | Error
      mask TypeOptions adder_imp: Fabric | DSP48 | Behavioural
  invert{1..9} (9 alike) : xbsIndex_r4/Inverter  en=off  latency=0  dbl_ovrd=off  block_type=inv
  slice1 : xbsIndex_r4/Slice  nbits=1  boolean_output=on  mode=Upper Bit Location + Width  bit1=0  base1=MSB of Input  bit0=0  base0=LSB of Input  dbl_ovrd=off  block_type=slice
  slice2 : xbsIndex_r4/Slice  nbits=1  boolean_output=on  mode=Upper Bit Location + Width  bit1=-1  base1=MSB of Input  bit0=0  base0=LSB of Input  dbl_ovrd=off  block_type=slice
  slice3 : xbsIndex_r4/Slice  nbits=1  boolean_output=on  mode=Upper Bit Location + Width  bit1=-2  base1=MSB of Input  bit0=0  base0=LSB of Input  dbl_ovrd=off  block_type=slice
  slice4 : xbsIndex_r4/Slice  nbits=1  boolean_output=on  mode=Upper Bit Location + Width  bit1=-3  base1=MSB of Input  bit0=0  base0=LSB of Input  dbl_ovrd=off  block_type=slice
  slice5 : xbsIndex_r4/Slice  nbits=1  boolean_output=on  mode=Upper Bit Location + Width  bit1=-4  base1=MSB of Input  bit0=0  base0=LSB of Input  dbl_ovrd=off  block_type=slice
  slice6 : xbsIndex_r4/Slice  nbits=1  boolean_output=on  mode=Upper Bit Location + Width  bit1=-5  base1=MSB of Input  bit0=0  base0=LSB of Input  dbl_ovrd=off  block_type=slice
  slice7 : xbsIndex_r4/Slice  nbits=1  boolean_output=on  mode=Upper Bit Location + Width  bit1=-6  base1=MSB of Input  bit0=0  base0=LSB of Input  dbl_ovrd=off  block_type=slice
  slice8 : xbsIndex_r4/Slice  nbits=1  boolean_output=on  mode=Upper Bit Location + Width  bit1=-7  base1=MSB of Input  bit0=0  base0=LSB of Input  dbl_ovrd=off  block_type=slice
  slice9 : xbsIndex_r4/Slice  nbits=1  boolean_output=on  mode=Upper Bit Location + Width  bit1=-8  base1=MSB of Input  bit0=0  base0=LSB of Input  dbl_ovrd=off  block_type=slice
  dout : Outport
  of : Outport  Port=2
  wires:
  din/1 -> convert/1(in), slice1/1, slice2/1, slice3/1, slice4/1, slice5/1, slice6/1, slice7/1, slice8/1, slice9/1
  convert/1(out) -> dout/1
  slice1/1 -> all_1s/1, invert1/1
  invert1/1 -> all_0s/1
  slice2/1 -> all_1s/2, invert2/1
  invert2/1 -> all_0s/2
  slice3/1 -> all_1s/3, invert3/1
  invert3/1 -> all_0s/3
  slice4/1 -> all_1s/4, invert4/1
  invert4/1 -> all_0s/4
  slice5/1 -> all_1s/5, invert5/1
  invert5/1 -> all_0s/5
  slice6/1 -> all_1s/6, invert6/1
  invert6/1 -> all_0s/6
  slice7/1 -> all_1s/7, invert7/1
  invert7/1 -> all_0s/7
  slice8/1 -> all_1s/8, invert8/1
  invert8/1 -> all_0s/8
  slice9/1 -> all_1s/9, invert9/1
  invert9/1 -> all_0s/9
  all_0s/1 -> and/1
  all_1s/1 -> and/2
  and/1 -> of/1
